simulink model "ControlMecCL"  (R2021a)
settings: Solver=VariableStepAuto  StartTime=0.0  StopTime=15  RelTol=1e-3
undefined symbols (not defined in the file): Dm, Dp, Dt, g, Jeq, Jp, k1, k2, k3, k4, km, kp, kv, Lm, Mb, Rm, thetaRef
settings Model: Creator=y.briere  LastModifiedBy=fades
settings SolverCC: AlgebraicLoopSolver=TrustRegion
settings DataIOCC: InitialState=[]  LoadInitialState=on  ReturnWorkspaceOutputs=off
settings DebuggingCC: SFMachineParentedDataDiag=warning  ArithmeticOperatorsInVariantConditions=warning
settings SFSimCC: CustomCodeUndefinedFunction=UseInterfaceOnly

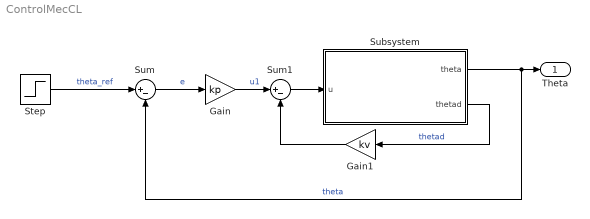
== system ControlMecCL ==
  Gain : Gain  Gain=kp
  Gain1 : Gain  Gain=kv
  Step : Step  Time=0  After=thetaRef*pi/180  SampleTime=0
  Subsystem : Subsystem
  Sum : Sum  Inputs=|+-
  Sum1 : Sum  Inputs=|+-
  Theta : Outport  VectorParamsAs1DForOutWhenUnconnected=off
  wires:
  Subsystem/1(theta) -> Sum/2, Theta/1  "theta"
  Step/1 -> Sum/1  "theta_ref"
  Sum/1 -> Gain/1  "e"
  Gain/1 -> Sum1/1  "u1"
  Sum1/1 -> Subsystem/1(u)
  Subsystem/2(thetad) -> Gain1/1  "thetad"
  Gain1/1 -> Sum1/2

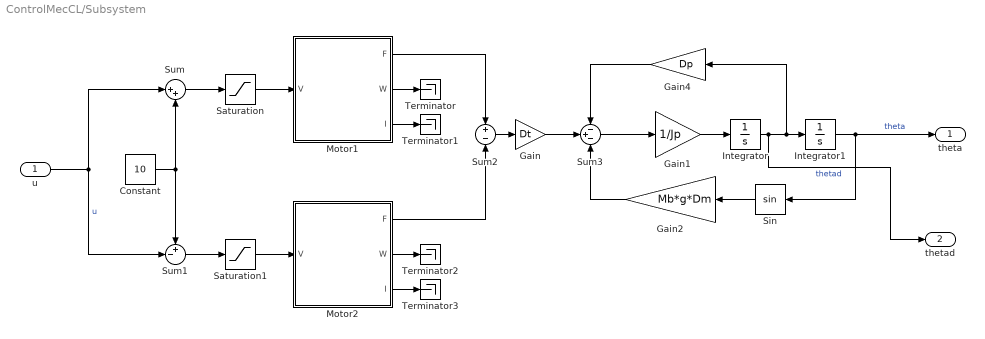
== system ControlMecCL/Subsystem ==
  u : Inport
  Constant : Constant  Value=10
  Gain : Gain  Gain=Dt
  Gain1 : Gain  Gain=1/Jp
  Gain2 : Gain  Gain=Mb*g*Dm
  Gain4 : Gain  Gain=Dp
  Integrator : Integrator
  Integrator1 : Integrator
  Motor1 : Subsystem
  Motor2 : Subsystem
  Saturation : Saturate  UpperLimit=24  LowerLimit=-24
  Saturation1 : Saturate  UpperLimit=24  LowerLimit=-24
  Sin : Trigonometry
  Sum : Sum  Inputs=|++
  Sum1 : Sum  Inputs=+-|
  Sum2 : Sum  Inputs=+-
  Sum3 : Sum  Inputs=-+-
  Terminator{,1..3} (4 alike) : Terminator
  theta : Outport  VectorParamsAs1DForOutWhenUnconnected=off
  thetad : Outport  Port=2  VectorParamsAs1DForOutWhenUnconnected=off
  wires:
  Sum2/1 -> Gain/1
  u/1 -> Sum1/2, Sum/1  "u"
  Motor1/2(W) -> Terminator/1
  Constant/1 -> Sum1/1, Sum/2
  Motor1/3(I) -> Terminator1/1
  Motor2/3(I) -> Terminator3/1
  Integrator/1 -> thetad/1, Gain4/1, Integrator1/1  "thetad"
  Integrator1/1 -> theta/1, Sin/1  "theta"
  Motor2/2(W) -> Terminator2/1
  Sum/1 -> Saturation/1
  Sum3/1 -> Gain1/1
  Gain4/1 -> Sum3/1
  Gain/1 -> Sum3/2
  Sum1/1 -> Saturation1/1
  Motor2/1(F) -> Sum2/2
  Gain1/1 -> Integrator/1
  Motor1/1(F) -> Sum2/1
  Sin/1 -> Gain2/1
  Gain2/1 -> Sum3/3
  Saturation/1 -> Motor1/1(V)
  Saturation1/1 -> Motor2/1(V)

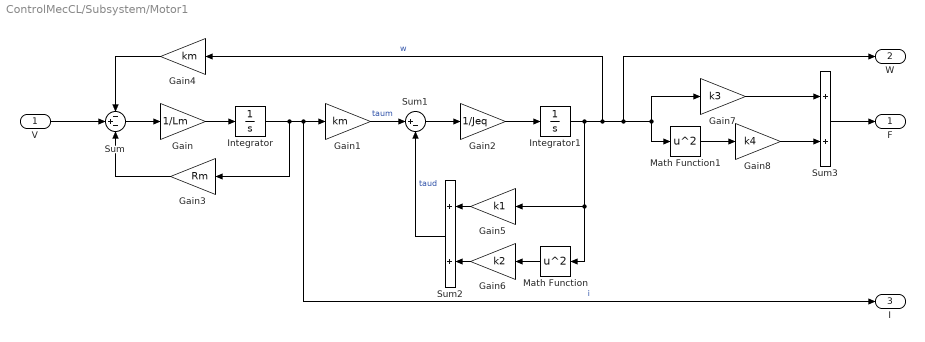
== system ControlMecCL/Subsystem/Motor1 ==
  V : Inport
  Gain : Gain  Gain=1/Lm
  Gain1 : Gain  Gain=km
  Gain2 : Gain  Gain=1/Jeq
  Gain3 : Gain  Gain=Rm
  Gain4 : Gain  Gain=km
  Gain5 : Gain  Gain=k1
  Gain6 : Gain  Gain=k2
  Gain7 : Gain  Gain=k3
  Gain8 : Gain  Gain=k4
  Integrator : Integrator
  Integrator1 : Integrator
  Math Function : Math  Operator=square  SignedPower=on  SaturateOnIntegerOverflow=on
  Math Function1 : Math  Operator=square  SignedPower=on  SaturateOnIntegerOverflow=on
  Sum : Sum  Inputs=-+-
  Sum1 : Sum  Inputs=|+-
  Sum2 : Sum
  Sum3 : Sum
  F : Outport  VectorParamsAs1DForOutWhenUnconnected=off
  W : Outport  Port=2  VectorParamsAs1DForOutWhenUnconnected=off
  I : Outport  Port=3  VectorParamsAs1DForOutWhenUnconnected=off
  wires:
  Gain5/1 -> Sum2/1
  Sum3/1 -> F/1
  Gain8/1 -> Sum3/2
  Math Function/1 -> Gain6/1
  Gain4/1 -> Sum/1
  Gain/1 -> Integrator/1
  Math Function1/1 -> Gain8/1
  Sum1/1 -> Gain2/1
  Gain6/1 -> Sum2/2
  Sum2/1 -> Sum1/2  "taud"
  Integrator/1 -> I/1, Gain1/1, Gain3/1  "i"
  Sum/1 -> Gain/1
  Gain7/1 -> Sum3/1
  Integrator1/1 -> Gain5/1, Math Function/1, W/1, Gain7/1, Math Function1/1, Gain4/1  "w"
  Gain3/1 -> Sum/3
  Gain1/1 -> Sum1/1  "taum"
  Gain2/1 -> Integrator1/1
  V/1 -> Sum/2

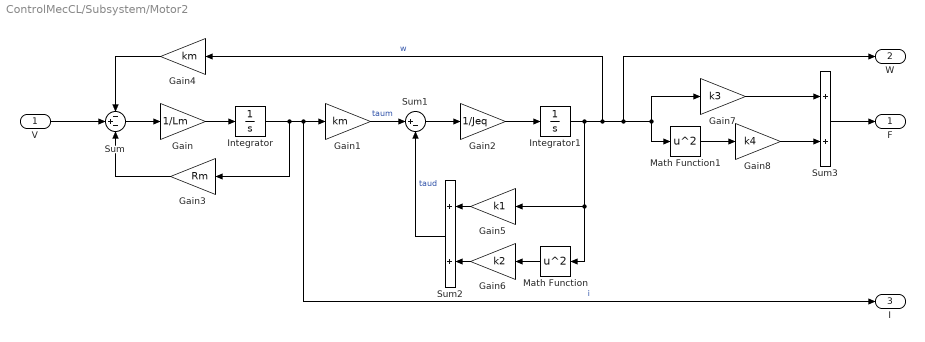
== system ControlMecCL/Subsystem/Motor2 ==
  V : Inport
  Gain : Gain  Gain=1/Lm
  Gain1 : Gain  Gain=km
  Gain2 : Gain  Gain=1/Jeq
  Gain3 : Gain  Gain=Rm
  Gain4 : Gain  Gain=km
  Gain5 : Gain  Gain=k1
  Gain6 : Gain  Gain=k2
  Gain7 : Gain  Gain=k3
  Gain8 : Gain  Gain=k4
  Integrator : Integrator
  Integrator1 : Integrator
  Math Function : Math  Operator=square  SignedPower=on  SaturateOnIntegerOverflow=on
  Math Function1 : Math  Operator=square  SignedPower=on  SaturateOnIntegerOverflow=on
  Sum : Sum  Inputs=-+-
  Sum1 : Sum  Inputs=|+-
  Sum2 : Sum
  Sum3 : Sum
  F : Outport  VectorParamsAs1DForOutWhenUnconnected=off
  W : Outport  Port=2  VectorParamsAs1DForOutWhenUnconnected=off
  I : Outport  Port=3  VectorParamsAs1DForOutWhenUnconnected=off
  wires:
  V/1 -> Sum/2
  Gain2/1 -> Integrator1/1
  Gain1/1 -> Sum1/1  "taum"
  Gain3/1 -> Sum/3
  Integrator1/1 -> Gain4/1, Math Function1/1, Gain7/1, W/1, Math Function/1, Gain5/1  "w"
  Gain7/1 -> Sum3/1
  Sum/1 -> Gain/1
  Integrator/1 -> Gain3/1, Gain1/1, I/1  "i"
  Sum2/1 -> Sum1/2  "taud"
  Gain6/1 -> Sum2/2
  Sum1/1 -> Gain2/1
  Math Function1/1 -> Gain8/1
  Gain/1 -> Integrator/1
  Gain4/1 -> Sum/1
  Math Function/1 -> Gain6/1
  Gain8/1 -> Sum3/2
  Sum3/1 -> F/1
  Gain5/1 -> Sum2/1
